simulink model "surekliModel_2022"  (R2022b)
settings: Solver=VariableStepAuto  StartTime=0.0  StopTime=5  RelTol=1e-3
values from neighbouring files (symbols this model uses):
  b = 0.000023873    (= 2.3873e-05)    [variables.m]
  J = 0.0000023    (= 2.3e-06)    [variables.m]
  kd = 4.5451e-08    [calculations.m]
  ke = 0.0000219    (= 2.19e-05)    [variables.m]
  ki = 62.1893    [calculations.m]
  kp = 1.38 * 1000    (= 1380)    [calculations.m]
  kt = 0.0000217    (= 2.17e-05)    [variables.m]
  L = 0.000113    [variables.m]
  R = 0.199    [variables.m]
  Y1 = x7 + x6 + (x5 + x3 + x2)/(etaWG)    (= 2.3434762323e-06)    [variables.m]
  Y2 = x4/(etaWG)    (= 0.00104761904762)    [variables.m]
  Y3 = x1/(etaWG)    (= 7.68395443415e-05)    [variables.m]
libraries: slpidlib x1
settings Model: LastModifiedBy=lenovo
settings OptimizationCC: ReuseModelBlockBuffer=on
settings RTWCC: GPUComputeCapability=5.0

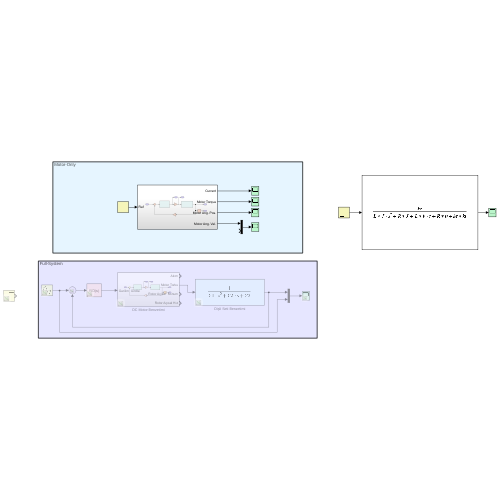
[thumbnail: Simulink's stored preview of the top-level diagram]
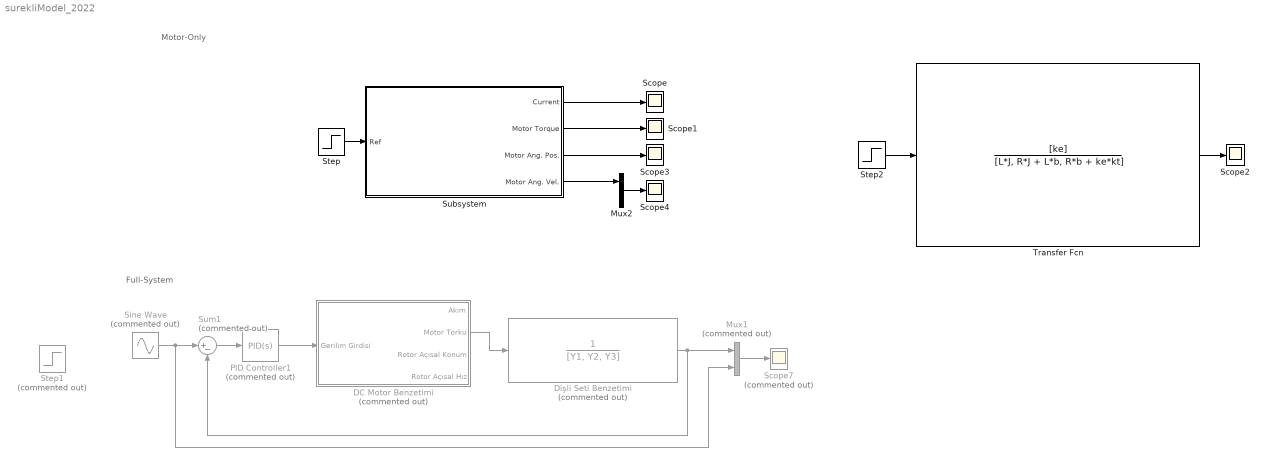
== system surekliModel_2022 ==
  note: Full-System
  note: Motor-Only
  DC Motor Benzetimi : Subsystem  Commented=on
  Dişli Seti Benzetimi : TransferFcn  Commented=on  Denominator=[Y1, Y2, Y3]
  Mux1 : Mux  Commented=on  Inputs=2
  Mux2 : Mux  Inputs=2
  PID Controller1 : slpidlib/PID Controller  Commented=on  Controller=PID  Form=Parallel  TimeDomain=Continuous-time  UseExternalTs=off  SampleTime=-1  IntegratorMethod=Forward Euler  FilterMethod=Forward Euler  ControllerParametersSource=internal  P=kp  I=ki  UseKiTs=off  D=kd  N=147.580492826738  UseFilter=on  TunerSelectOption=Transfer Function Based (PID Tuner App)  InitialConditionSource=internal  InitialConditionForIntegrator=0  InitialConditionForFilter=0  DifferentiatorICPrevScaledInput=0  ExternalReset=none  TrackingMode=off  Kt=1  LimitOutput=off  SatLimitsSource=internal  UpperSaturationLimit=inf  LowerSaturationLimit=-inf  LinearizeAsGain=on  AntiWindupMode=none  Kb=1  LimitIntegrator=off  UpperIntegratorSaturationLimit=inf  LowerIntegratorSaturationLimit=-inf  POutMin=[]  POutMax=[]  IOutMin=[]  IOutMax=[]  DOutMin=[]  DOutMax=[]  NOutMin=[]  NOutMax=[]  SumOutMin=[]  SumOutMax=[]  SaturationOutMin=[]  SaturationOutMax=[]  PParamMin=[]  PParamMax=[]  IParamMin=[]  IParamMax=[]  DParamMin=[]  DParamMax=[]  NParamMin=[]  NParamMax=[]  KbParamMin=[]  KbParamMax=[]  KtParamMin=[]  KtParamMax=[]  KbOutMin=[]  KbOutMax=[]  KtOutMin=[]  KtOutMax=[]  IntegratorOutMin=[]  IntegratorOutMax=[]  FilterOutMin=[]  FilterOutMax=[]  SumI1OutMin=[]  SumI1OutMax=[]  SumI2OutMin=[]  SumI2OutMax=[]  SumI3OutMin=[]  SumI3OutMax=[]  SumI4OutMin=[]  SumI4OutMax=[]  SumDOutMin=[]  SumDOutMax=[]  DifferentiatorOutMin=[]  DifferentiatorOutMax=[]  FilterDiffOutCoefMin=[]  FilterDiffOutCoefMax=[]  ReciprocalOutMin=[]  ReciprocalOutMax=[]  SumDenOutMin=[]  SumDenOutMax=[]  SumNumOutMin=[]  SumNumOutMax=[]  DivideOutMin=[]  DivideOutMax=[]  UdiffTsProdOutMin=[]  UdiffTsProdOutMax=[]  NTsProdOutMin=[]  NTsProdOutMax=[]  UintegralTsProdOutMin=[]  UintegralTsProdOutMax=[]  UngainTsProdOutMin=[]  UngainTsProdOutMax=[]  ClampingZeroOutDataTypeStr=Inherit: Inherit via back propagation  ClampingZeroOutMin=[]  ClampingZeroOutMax=[]  FilterDenConstantOutDataTypeStr=Inherit: Inherit via back propagation  FilterDenConstantOutMin=[]  FilterDenConstantOutMax=[]  PCopyOutDataTypeStr=Inherit: Inherit via back propagation  PCopyOutMin=[]  PCopyOutMax=[]  NCopyOutDataTypeStr=Inherit: Inherit via back propagation  NCopyOutMin=[]  NCopyOutMax=[]  IntegratorContinuousStateAttributes=''  IntegratorStateMustResolveToSignalObject=off  IntegratorRTWStateStorageClass=Auto  FilterContinuousStateAttributes=''  FilterStateMustResolveToSignalObject=off  FilterRTWStateStorageClass=Auto  ParallelPVariant=InternalParameters  IdealPVariant=Disabled  IVariant=InternalParameters  DVariant=InternalParameters  IntegratorVariant=Continuous  SatVariant=Disabled  AWVariant=Passthrough  PCopyVariant=Disabled  TRVariant=Disabled  FdbkBlocksVariant=Forward  IdealPFdbkVariant=Disabled  SatFdbkVariant=Disabled  DerivativeFilterVariant=ContFilter  NVariant=InternalParameters  NCopyVariant=Disabled  FilterICVariant=InternalICsFilter  IntegratorICVariant=InternalICs  ExternalResetVariant=Disabled  TRSumVariant=Passthrough  SumFdbkVariant=Disabled  SumVariant=Sum_PID  TsampFilterVariant=InternalTs  TsampNgainVariant=Passthrough  TsampIntegralVariant=Passthrough  ExternalSaturationOutDataTypeStr=Inherit: Same as second input
  Scope{,1..4} (5 alike) : Scope
  Scope7 : Scope  Commented=on
  Sine Wave : Sin  Commented=on  Frequency=2.5  SampleTime=0
  Step : Step  Time=0  After=10  SampleTime=0
  Step1 : Step  Commented=on  Time=0  After=10  SampleTime=0
  Step2 : Step  Time=0  After=10  SampleTime=0
  Subsystem : Subsystem
  Sum1 : Sum  Commented=on  Inputs=|+-
  Transfer Fcn : TransferFcn  Numerator=[ke]  Denominator=[L*J, R*J + L*b, R*b + ke*kt]
  wires:
  Subsystem/1(Current) -> Scope/1
  Subsystem/2(Motor Torque) -> Scope1/1
  Subsystem/3(Motor Ang. Pos.) -> Scope3/1
  Subsystem/4(Motor Ang. Vel.) -> Mux2/1
  Sum1/1 -> PID Controller1/1
  Sine Wave/1 -> Mux1/2, Sum1/1
  Mux2/1 -> Scope4/1
  PID Controller1/1 -> DC Motor Benzetimi/1(Gerilim Girdisi)
  Dişli Seti Benzetimi/1 -> Mux1/1, Sum1/2
  Mux1/1 -> Scope7/1
  DC Motor Benzetimi/2(Motor Torku) -> Dişli Seti Benzetimi/1
  Step2/1 -> Transfer Fcn/1
  Transfer Fcn/1 -> Scope2/1
  Step/1 -> Subsystem/1(Ref)

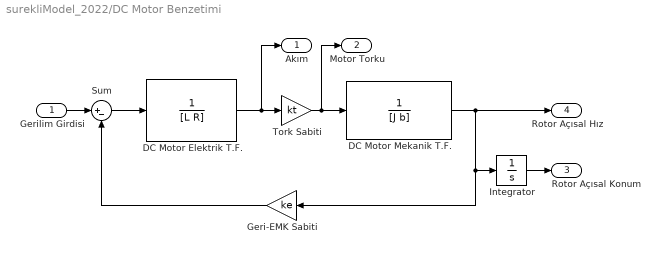
== system surekliModel_2022/DC Motor Benzetimi ==
  Gerilim Girdisi : Inport
  DC Motor Elektrik T.F. : TransferFcn  Denominator=[L R]
  DC Motor Mekanik T.F. : TransferFcn  Denominator=[J b]
  Geri-EMK Sabiti : Gain  Gain=ke
  Integrator : Integrator
  Sum : Sum  Inputs=|+-
  Tork Sabiti : Gain  Gain=kt
  Akım : Outport
  Motor Torku : Outport  Port=2
  Rotor Açısal Konum : Outport  Port=3
  Rotor Açısal Hız : Outport  Port=4
  wires:
  Tork Sabiti/1 -> Motor Torku/1, DC Motor Mekanik T.F./1
  Sum/1 -> DC Motor Elektrik T.F./1
  Geri-EMK Sabiti/1 -> Sum/2
  Gerilim Girdisi/1 -> Sum/1
  DC Motor Elektrik T.F./1 -> Akım/1, Tork Sabiti/1
  Integrator/1 -> Rotor Açısal Konum/1
  DC Motor Mekanik T.F./1 -> Integrator/1, Geri-EMK Sabiti/1, Rotor Açısal Hız/1

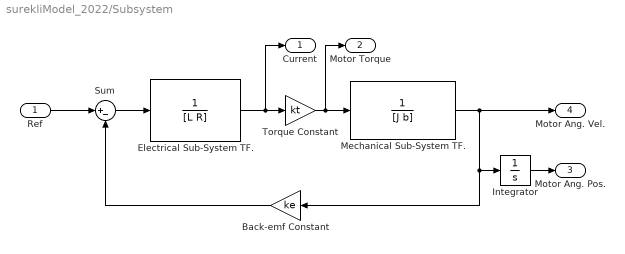
== system surekliModel_2022/Subsystem ==
  Ref : Inport
  "Back-emf Constant " : Gain  Gain=ke
  Electrical Sub-System TF. : TransferFcn  Denominator=[L R]
  Integrator : Integrator
  Mechanical Sub-System TF. : TransferFcn  Denominator=[J b]
  Sum : Sum  Inputs=|+-
  Torque Constant : Gain  Gain=kt
  Current : Outport
  Motor Torque : Outport  Port=2
  Motor Ang. Pos. : Outport  Port=3
  Motor Ang. Vel. : Outport  Port=4
  wires:
  Torque Constant/1 -> Motor Torque/1, Mechanical Sub-System TF./1
  Sum/1 -> Electrical Sub-System TF./1
  "Back-emf Constant "/1 -> Sum/2
  Ref/1 -> Sum/1
  Electrical Sub-System TF./1 -> Current/1, Torque Constant/1
  Integrator/1 -> Motor Ang. Pos./1
  Mechanical Sub-System TF./1 -> Integrator/1, "Back-emf Constant "/1, Motor Ang. Vel./1
